simulink model "circles"  (Simulink 4.00)
settings: Solver=ode45  StartTime=0.0  StopTime=4*pi  MaxStep=0.001*pi  RelTol=1e-3
settings Model: LastModifiedBy=acataldo

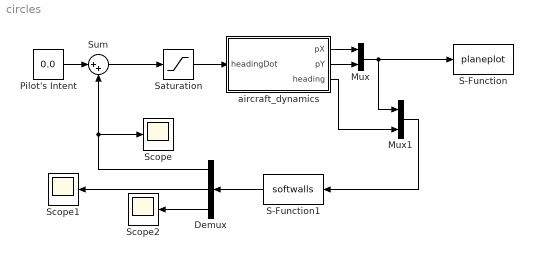
== system circles ==
  Demux : Demux  Orientation=left  Outputs=3  BusSelectionMode=off
  Mux : Mux  Inputs=2
  Mux1 : Mux  Inputs=2
  Pilot's Intent : Constant  Value=0.0
  S-Function : S-Function  FunctionName=planeplot  PortCounts=[]  SFunctionModules=''
  S-Function1 : S-Function  Orientation=left  FunctionName=softwalls  PortCounts=[]  SFunctionModules=''
  Saturation : Saturate  UpperLimit=1.0 / 0.15  LowerLimit=-1.0 / 0.15  LinearizeAsGain=on
  Scope : Scope
      settings: TimeRange=auto  YMin=-250  YMax=300  SaveToWorkspace=off  SaveName=ScopeData  LimitDataPoints=on  MaxDataPoints=5000
  Scope1 : Scope
      settings: TimeRange=auto  YMin=-5  YMax=5  SaveToWorkspace=off  LimitDataPoints=on  MaxDataPoints=5000
  Scope2 : Scope
      settings: TimeRange=auto  YMin=-5  YMax=5  SaveToWorkspace=off  SaveName=ScopeData2  LimitDataPoints=on  MaxDataPoints=5000
  Sum : Sum  Inputs=|++  SaturateOnIntegerOverflow=on
  aircraft_dynamics : Subsystem  TreatAsAtomicUnit=on
      settings: RTWFcnNameOpts=Auto  RTWFileNameOpts=Auto
  wires:
  Pilot's Intent/1 -> Sum/1
  aircraft_dynamics/1(pX) -> Mux/1
  aircraft_dynamics/2(pY) -> Mux/2
  Mux/1 -> S-Function/1, Mux1/1
  aircraft_dynamics/3(heading) -> Mux1/2
  Mux1/1 -> S-Function1/1
  Sum/1 -> Saturation/1
  Saturation/1 -> aircraft_dynamics/1(headingDot)
  S-Function1/1 -> Demux/1
  Demux/1 -> Scope/1, Sum/2
  Demux/2 -> Scope1/1
  Demux/3 -> Scope2/1

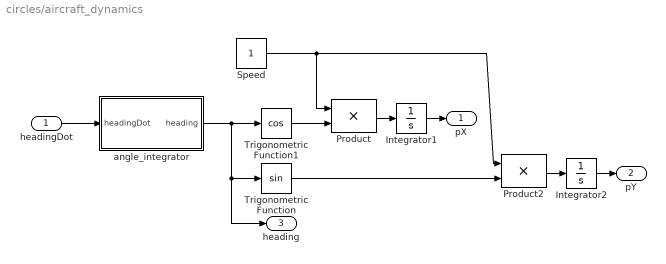
== system circles/aircraft_dynamics ==
  headingDot : Inport  Port=1  LatchInput=off
  Integrator1 : Integrator  ExternalReset=none  InitialConditionSource=internal  InitialCondition=1  LimitOutput=off  UpperSaturationLimit=inf  LowerSaturationLimit=-inf  ShowSaturationPort=off  ShowStatePort=off  AbsoluteTolerance=auto
      settings: AttributesFormatString=initial_X = %<InitialCondition>
  Integrator2 : Integrator  ExternalReset=none  InitialConditionSource=internal  InitialCondition=-1  LimitOutput=off  UpperSaturationLimit=inf  LowerSaturationLimit=-inf  ShowSaturationPort=off  ShowStatePort=off  AbsoluteTolerance=auto
      settings: AttributesFormatString=initial_Y = %<InitialCondition>
  Product : Product  Inputs=2  Multiplication=Element-wise(.*)  SaturateOnIntegerOverflow=on
  Product2 : Product  Inputs=2  Multiplication=Element-wise(.*)  SaturateOnIntegerOverflow=on
  Speed : Constant  Value=1
  Trigonometric Function : Trigonometry  Operator=sin  OutputSignalType=auto
  Trigonometric Function1 : Trigonometry  Operator=cos  OutputSignalType=auto
  angle_integrator : Subsystem  TreatAsAtomicUnit=on
      settings: RTWFcnNameOpts=Auto  RTWFileNameOpts=Auto
  pX : Outport  Port=1
  pY : Outport  Port=2
  heading : Outport  Port=3
  wires:
  Speed/1 -> Product/1, Product2/1
  angle_integrator/1(heading) -> Trigonometric Function1/1, Trigonometric Function/1, heading/1
  Trigonometric Function1/1 -> Product/2
  Trigonometric Function/1 -> Product2/2
  Product/1 -> Integrator1/1
  Integrator1/1 -> pX/1
  Product2/1 -> Integrator2/1
  Integrator2/1 -> pY/1
  headingDot/1 -> angle_integrator/1(headingDot)

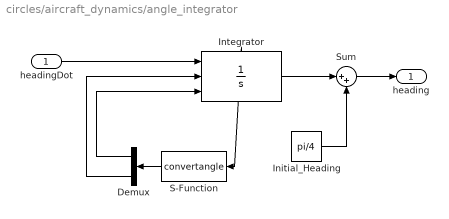
== system circles/aircraft_dynamics/angle_integrator ==
  headingDot : Inport  Port=1  LatchInput=off
  Demux : Demux  Orientation=left  Outputs=2  BusSelectionMode=off
  Initial_Heading : Constant  Value=pi/4
  Integrator : Integrator  ExternalReset=level  InitialConditionSource=external  InitialCondition=0  LimitOutput=off  UpperSaturationLimit=inf  LowerSaturationLimit=-inf  ShowSaturationPort=off  ShowStatePort=on  AbsoluteTolerance=auto
  S-Function : S-Function  Orientation=left  FunctionName=convertangle  PortCounts=[]  SFunctionModules=''
  Sum : Sum  Inputs=|++  SaturateOnIntegerOverflow=on
  heading : Outport  Port=1
  wires:
  headingDot/1 -> Integrator/1
  S-Function/1 -> Demux/1
  Demux/1 -> Integrator/3
  Demux/2 -> Integrator/2
  Integrator/State -> S-Function/1
  Integrator/1 -> Sum/1
  Initial_Heading/1 -> Sum/2
  Sum/1 -> heading/1
